simulink model "Expt_4_3"  (R2018a)
settings: Solver=VariableStepAuto  StartTime=0.0  StopTime=10.0  RelTol=1e-3
libraries: simulink x1
settings Model: Creator=HP  LastModifiedBy=HP

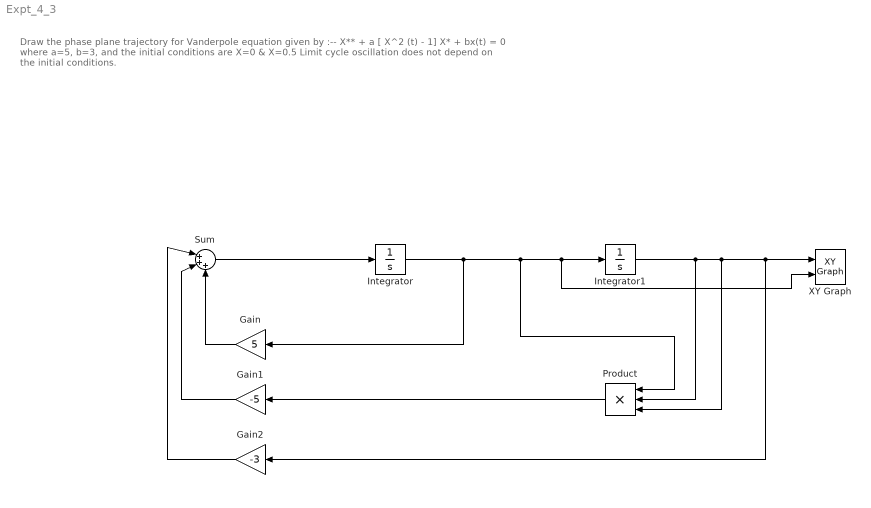
== system Expt_4_3 ==
  note: Draw the phase plane trajectory for Vanderpole equation given by :--
      |
      | X** + a [ X^2 (t) - 1] X* + bx(t) = 0 where a=5, b=3, and the initial conditions are X=0 & X=0.5
      |
      | Limit cycle oscillation does not depend on the initial conditions.
  Gain : Gain  Gain=5
  Gain1 : Gain  Gain=-5
  Gain2 : Gain  Gain=-3
  Integrator : Integrator  InitialCondition=1
  Integrator1 : Integrator  InitialCondition=1
  Product : Product  Inputs=3
  Sum : Sum  Inputs=|+++
  XY Graph : simulink/Sinks/XY Graph  xmin=-10  xmax=10  ymin=-10  ymax=10  st=-1
  wires:
  Integrator1/1 -> Product/2, Product/3, XY Graph/1, Gain2/1
  Gain/1 -> Sum/3
  Gain1/1 -> Sum/2
  Gain2/1 -> Sum/1
  Product/1 -> Gain1/1
  Sum/1 -> Integrator/1
  Integrator/1 -> Gain/1, Product/1, XY Graph/2, Integrator1/1
